simulink model "msd_model"  (R2019b)
settings: Solver=VariableStepAuto  StartTime=0.0  StopTime=20  RelTol=1e-3
values from neighbouring files (symbols this model uses):
  b = 1    [MainScript.m]
  k = 1    [MainScript.m]
  m = 1    [MainScript.m]
  stepf = 1    [MainScript.m]
  stepi = 0    [MainScript.m]
  stept = 2    [MainScript.m]
  vel0 = 0    [MainScript.m]
  x0 = 0    [MainScript.m]
settings Model: Creator=mountj  LastModifiedBy=n9182250
settings DataIOCC: TimeSaveName=mytime

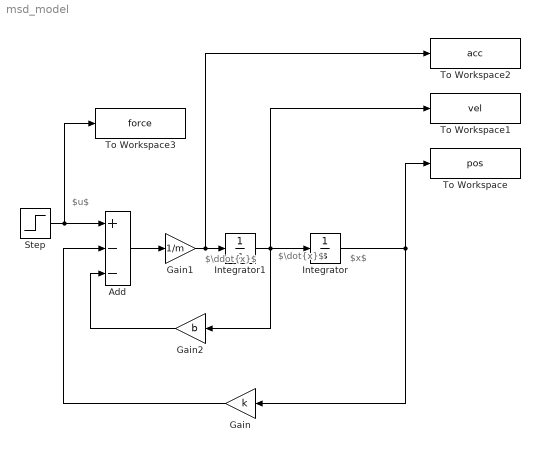
== system msd_model ==
  note: $\dot{x}$
  note: $x$
  note: $\ddot{x}$
  note: $u$
  Add : Sum  Inputs=+--
  Gain : Gain  Gain=k
  Gain1 : Gain  Gain=1/m
  Gain2 : Gain  Gain=b
  Integrator : Integrator  InitialCondition=x0
  Integrator1 : Integrator  InitialCondition=vel0
  Step : Step  Time=stept  Before=stepi  After=stepf  SampleTime=0
  To Workspace : ToWorkspace  VariableName=pos  SampleTime=-1
  To Workspace1 : ToWorkspace  VariableName=vel  SampleTime=-1
  To Workspace2 : ToWorkspace  VariableName=acc  SampleTime=-1
  To Workspace3 : ToWorkspace  VariableName=force  SampleTime=-1
  wires:
  Integrator1/1 -> To Workspace1/1, Gain2/1, Integrator/1
  Integrator/1 -> To Workspace/1, Gain/1
  Step/1 -> To Workspace3/1, Add/1
  Gain/1 -> Add/2
  Add/1 -> Gain1/1
  Gain1/1 -> To Workspace2/1, Integrator1/1
  Gain2/1 -> Add/3
